simulink model "pump_elastic_sim"  (R2020a)
settings: Solver=VariableStepAuto  StartTime=0.0  StopTime=10  RelTol=1e-3
values from neighbouring files (symbols this model uses):
  A = 0.3    [Shape_Function.m]
  l = 8    [Shape_Function.m]
  rho = 7833    [Shape_Function.m]
undefined symbols (not defined in the file or in its folder): Al, B, Cd, Cl, g, G1, G2, G3, G4, G5, G6, h, Jx, Jy, K, m, mu0, Nr, P1, P2, P3, P4, P5, P6, PHI12, PHI20, PHI4, phi_init, PHIc, PHIf, PHIr, qv_init, R, radius, Ss, theta_init, vqv_init, Vref, vx, w, xA, xB, xdot_ref, xe, yB, zA, zB, zi_rip
settings Model: Creator=adelina  LastModifiedBy=Federico

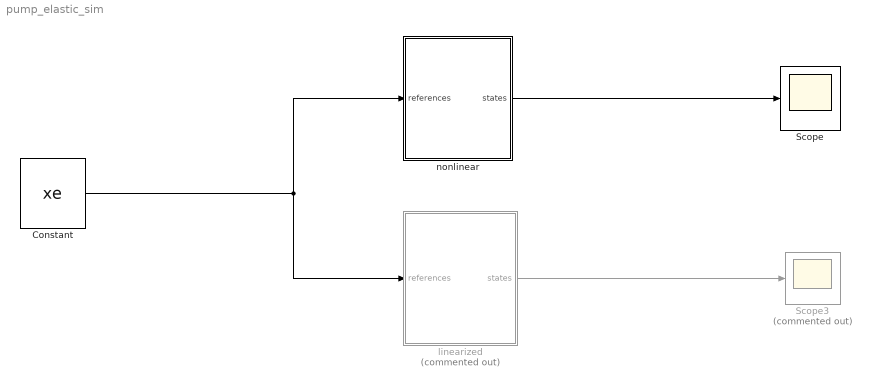
== system pump_elastic_sim ==
  Constant : Constant  Value=xe
  Scope : Scope
  Scope3 : Scope  Commented=on
  linearized : Subsystem  Commented=on
  nonlinear : Subsystem
  wires:
  linearized/1(states) -> Scope3/1
  nonlinear/1(states) -> Scope/1
  Constant/1 -> nonlinear/1(references), linearized/1(references)

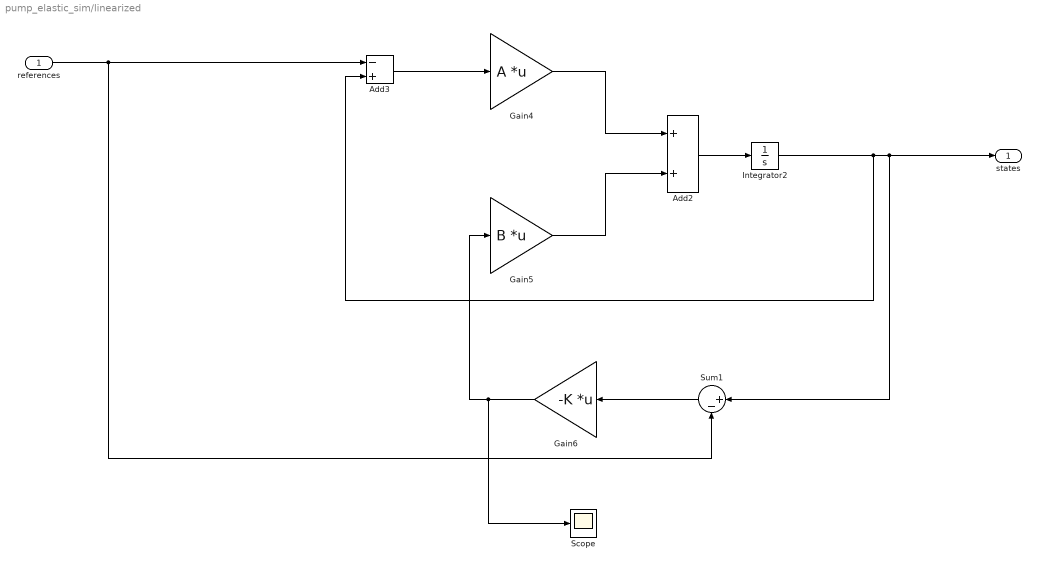
== system pump_elastic_sim/linearized ==
  references : Inport
  Add2 : Sum
  Add3 : Sum  Inputs=-+
  Gain4 : Gain  Gain=A  Multiplication=Matrix(K*u)
  Gain5 : Gain  Gain=B  Multiplication=Matrix(K*u)
  Gain6 : Gain  Gain=-K  Multiplication=Matrix(K*u)
  Integrator2 : Integrator  InitialCondition=[h;0;0;0;0;0;0;0;0;0;0;0]
  Scope : Scope
  Sum1 : Sum  Inputs=|+-
  states : Outport
  wires:
  Add2/1 -> Integrator2/1
  Gain5/1 -> Add2/2
  Gain6/1 -> Scope/1, Gain5/1
  Gain4/1 -> Add2/1
  Integrator2/1 -> states/1, Sum1/1, Add3/2
  Add3/1 -> Gain4/1
  references/1 -> Sum1/2, Add3/1
  Sum1/1 -> Gain6/1

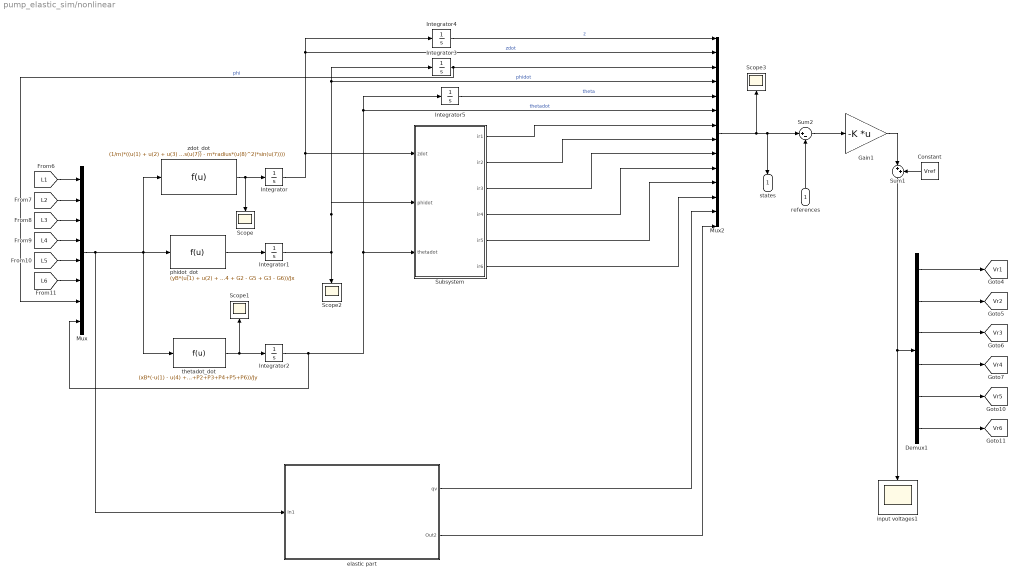
== system pump_elastic_sim/nonlinear ==
  references : Inport
  Constant : Constant  Value=Vref
  Demux1 : Demux  Outputs=6
  Gain1 : Gain  Gain=-K  Multiplication=Matrix(K*u)
  Integrator : Integrator
  Integrator1 : Integrator
  Integrator2 : Integrator
  Integrator3 : Integrator  InitialCondition=phi_init
  Integrator4 : Integrator  InitialCondition=h
  Integrator5 : Integrator  InitialCondition=theta_init
  Mux : Mux  Inputs=8
  Mux2 : Mux  Inputs=14
  Scope{,1..3} (4 alike) : Scope
  Subsystem : Subsystem
  Sum1 : Sum  Inputs=|++
  Sum2 : Sum  Inputs=|+-
  elastic part : Subsystem
  input voltages1 : Scope
  phidot_dot : Fcn  Expr=(yB*(u(1) + u(2) + u(3) - u(4) - u(5) - u(6)) + zB*(G1 - G4 + G2 - G5 + G3 - G6))/Jx
  thetadot_dot : Fcn  Expr=(xB*(-u(1) - u(4) + u(3) + u(6)) -zA*(rho*Ss*Cd/2)*(xdot_ref)^2+xA*(rho*Ss*Cl/2)*(xdot_ref)^2+zB*(P1+P2+P3+P4+P5+P6))/Jy
  zdot_dot : Fcn  Expr=(1/m)*((u(1) + u(2) + u(3) + u(4) + u(5) + u(6) - (rho*Ss*Cl/2)*(xdot_ref)^2 - m*g*cos(u(7)) - m*radius*(u(8)^2)*sin(u(7))))
  states : Outport
  tag scope: Vr1=global, Vr2=global, Vr3=global, Vr4=global, Vr5=global, Vr6=global
  wires:
  Mux/1 -> elastic part/1(In1), thetadot_dot/1, phidot_dot/1, zdot_dot/1
  zdot_dot/1 -> Scope/1, Integrator/1
  Integrator/1 -> Integrator4/1, Mux2/2, Subsystem/1(zdot)  "zdot"
  phidot_dot/1 -> Integrator1/1
  Integrator1/1 -> Scope2/1, Mux2/4, Integrator3/1, Subsystem/2(phidot)  "phidot"
  thetadot_dot/1 -> Integrator2/1, Scope1/1
  Integrator2/1 -> Mux2/6, Integrator5/1, Subsystem/3(thetadot), Mux/8  "thetadot"
  [L1] -> Mux/1
  [L2] -> Mux/2
  [L3] -> Mux/3
  [L4] -> Mux/4
  [L5] -> Mux/5
  [L6] -> Mux/6
  Integrator3/1 -> Mux2/3, Mux/7  "phi"
  Demux1/4 -> [Vr4]
  Demux1/3 -> [Vr3]
  Demux1/2 -> [Vr2]
  Demux1/1 -> [Vr1]
  Sum2/1 -> Gain1/1
  Demux1/5 -> [Vr5]
  Demux1/6 -> [Vr6]
  Integrator4/1 -> Mux2/1  "z"
  Integrator5/1 -> Mux2/5  "theta"
  Subsystem/1(ir1) -> Mux2/7
  Subsystem/2(ir2) -> Mux2/8
  Subsystem/3(ir3) -> Mux2/9
  Subsystem/4(ir4) -> Mux2/10
  Subsystem/5(ir5) -> Mux2/11
  Subsystem/6(ir6) -> Mux2/12
  Mux2/1 -> Scope3/1, states/1, Sum2/1
  elastic part/1(qv) -> Mux2/13
  elastic part/2(Out2) -> Mux2/14
  references/1 -> Sum2/2
  Gain1/1 -> Sum1/1
  Sum1/1 -> Demux1/1, input voltages1/1
  Constant/1 -> Sum1/2

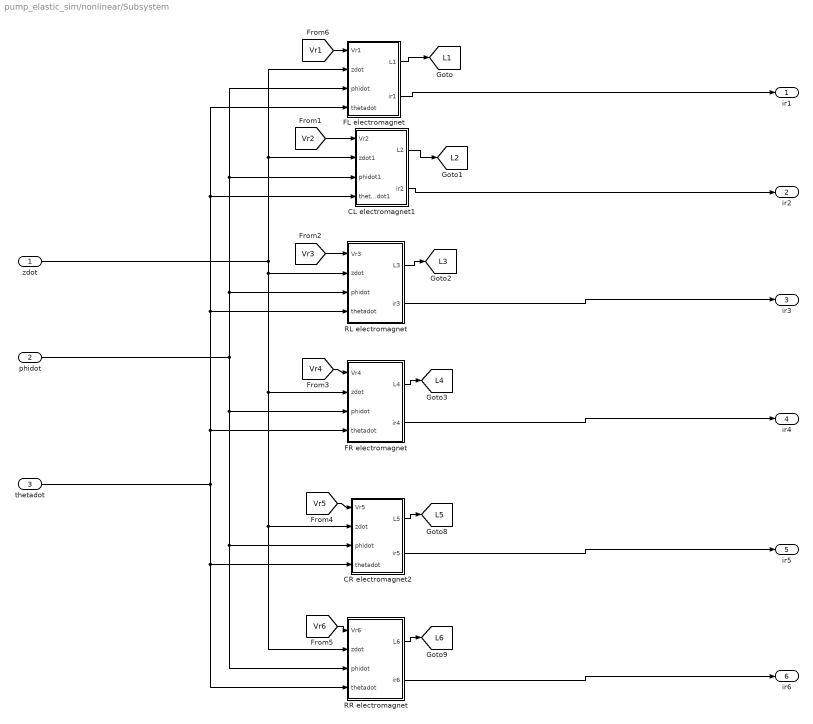
== system pump_elastic_sim/nonlinear/Subsystem ==
  zdot : Inport
  phidot : Inport  Port=2
  thetadot : Inport  Port=3
  CL electromagnet1 : Subsystem
  CR electromagnet2 : Subsystem
  FL electromagnet : Subsystem
  FR electromagnet : Subsystem
  RL electromagnet : Subsystem
  RR electromagnet : Subsystem
  ir1 : Outport
  ir2 : Outport  Port=2
  ir3 : Outport  Port=3
  ir4 : Outport  Port=4
  ir5 : Outport  Port=5
  ir6 : Outport  Port=6
  tag scope: L1=global, L2=global, L3=global, L4=global, L5=global, L6=global
  wires:
  CL electromagnet1/2(ir2) -> ir2/1
  [Vr3] -> RL electromagnet/1(Vr3)
  FR electromagnet/1(L4) -> [L4]
  CL electromagnet1/1(L2) -> [L2]
  FL electromagnet/1(L1) -> [L1]
  RR electromagnet/1(L6) -> [L6]
  CR electromagnet2/1(L5) -> [L5]
  [Vr6] -> RR electromagnet/1(Vr6)
  phidot/1 -> FR electromagnet/3(phidot), RR electromagnet/3(phidot), CR electromagnet2/3(phidot), FL electromagnet/3(phidot), CL electromagnet1/3(phidot1), RL electromagnet/3(phidot)
  [Vr4] -> FR electromagnet/1(Vr4)
  FR electromagnet/2(ir4) -> ir4/1
  zdot/1 -> CL electromagnet1/2(zdot1), FL electromagnet/2(zdot), RL electromagnet/2(zdot), FR electromagnet/2(zdot), RR electromagnet/2(zdot), CR electromagnet2/2(zdot)
  RL electromagnet/2(ir3) -> ir3/1
  FL electromagnet/2(ir1) -> ir1/1
  [Vr2] -> CL electromagnet1/1(Vr2)
  thetadot/1 -> RR electromagnet/4(thetadot), CR electromagnet2/4(thetadot), FL electromagnet/4(thetadot), CL electromagnet1/4(thetadot1), RL electromagnet/4(thetadot), FR electromagnet/4(thetadot)
  CR electromagnet2/2(ir5) -> ir5/1
  [Vr5] -> CR electromagnet2/1(Vr5)
  RR electromagnet/2(ir6) -> ir6/1
  RL electromagnet/1(L3) -> [L3]
  [Vr1] -> FL electromagnet/1(Vr1)

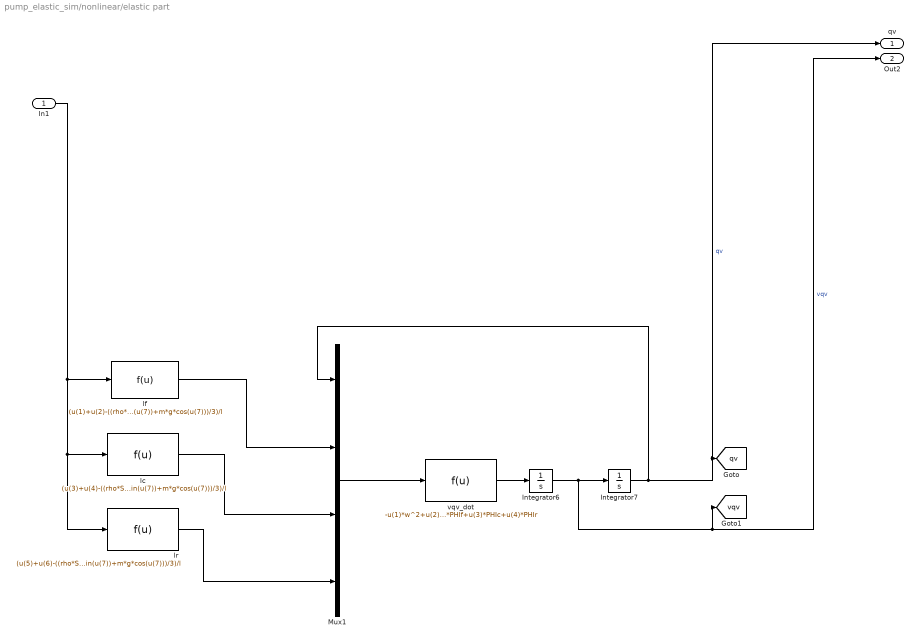
== system pump_elastic_sim/nonlinear/elastic part ==
  In1 : Inport
  Integrator6 : Integrator  InitialCondition=vqv_init
  Integrator7 : Integrator  InitialCondition=qv_init
  Mux1 : Mux
  lc : Fcn  Expr=(u(3)+u(4)-((rho*Ss*Cl/2)*(vx)^2+m*R*(u(8)^2)*sin(u(7))+m*g*cos(u(7)))/3)/l
  lf : Fcn  Expr=(u(1)+u(2)-((rho*Ss*Cl/2)*(vx)^2+m*R*(u(8)^2)*sin(u(7))+m*g*cos(u(7)))/3)/l
  lr : Fcn  Expr=(u(5)+u(6)-((rho*Ss*Cl/2)*(vx)^2+m*R*(u(8)^2)*sin(u(7))+m*g*cos(u(7)))/3)/l
  vqv_dot : Fcn  Expr=-u(1)*w^2+u(2)*PHIf+u(3)*PHIc+u(4)*PHIr
  qv : Outport
  Out2 : Outport  Port=2
  tag scope: qv=global, vqv=global
  wires:
  In1/1 -> lc/1, lr/1, lf/1
  Mux1/1 -> vqv_dot/1
  lf/1 -> Mux1/2
  vqv_dot/1 -> Integrator6/1
  Integrator7/1 -> qv/1, [qv], Mux1/1  "qv"
  lc/1 -> Mux1/3
  Integrator6/1 -> Out2/1, [vqv], Integrator7/1  "vqv"
  lr/1 -> Mux1/4

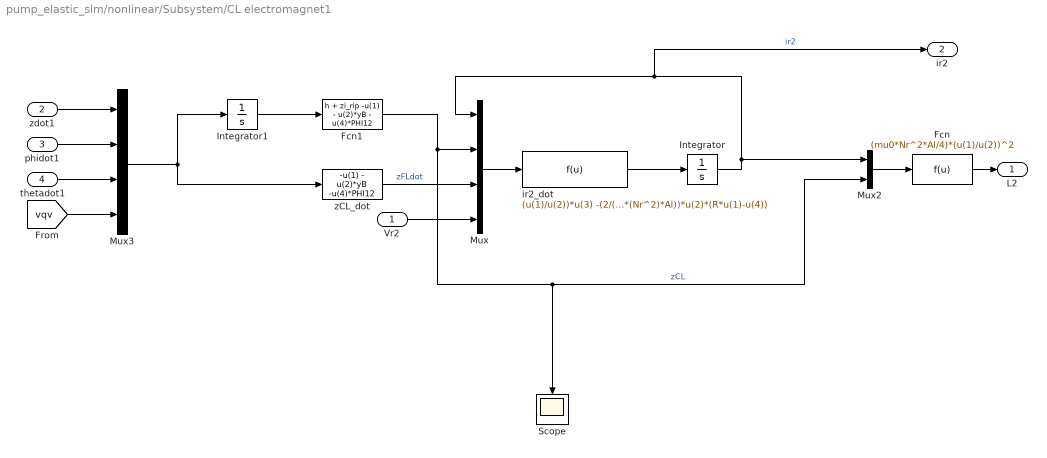
== system pump_elastic_sim/nonlinear/Subsystem/CL electromagnet1 ==
  Vr2 : Inport
  zdot1 : Inport  Port=2
  phidot1 : Inport  Port=3
  thetadot1 : Inport  Port=4
  Fcn : Fcn  Expr=(mu0*Nr^2*Al/4)*(u(1)/u(2))^2
  Fcn1 : Fcn  Expr=h + zi_rip -u(1) - u(2)*yB - u(4)*PHI12
  Integrator : Integrator
  Integrator1 : Integrator  InitialCondition=[h; phi_init; theta_init;qv_init]
  Mux : Mux
  Mux2 : Mux  Inputs=2
  Mux3 : Mux
  Scope : Scope
  ir2_dot : Fcn  Expr=(u(1)/u(2))*u(3) -(2/(mu0*(Nr^2)*Al))*u(2)*(R*u(1)-u(4))
  zCL_dot : Fcn  Expr=-u(1) - u(2)*yB -u(4)*PHI12
  L2 : Outport
  ir2 : Outport  Port=2
  wires:
  Mux/1 -> ir2_dot/1
  Vr2/1 -> Mux/4
  ir2_dot/1 -> Integrator/1
  Integrator/1 -> Mux2/1, ir2/1, Mux/1  "ir2"
  zCL_dot/1 -> Mux/3  "zFLdot"
  Fcn1/1 -> Scope/1, Mux2/2, Mux/2  "zCL"
  Mux2/1 -> Fcn/1
  Fcn/1 -> L2/1
  Integrator1/1 -> Fcn1/1
  thetadot1/1 -> Mux3/3
  phidot1/1 -> Mux3/2
  zdot1/1 -> Mux3/1
  [vqv] -> Mux3/4
  Mux3/1 -> zCL_dot/1, Integrator1/1

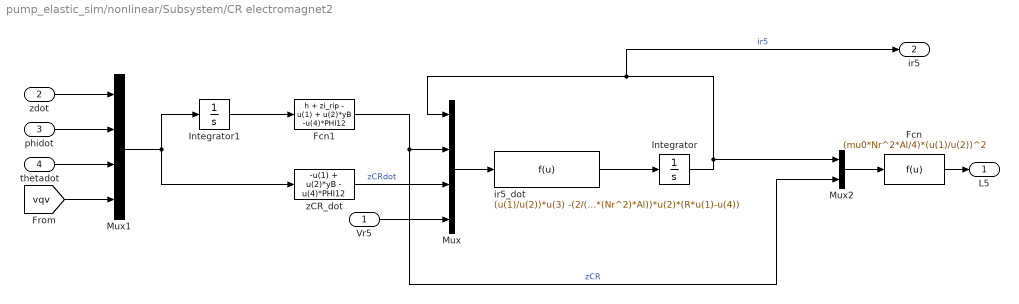
== system pump_elastic_sim/nonlinear/Subsystem/CR electromagnet2 ==
  Vr5 : Inport
  zdot : Inport  Port=2
  phidot : Inport  Port=3
  thetadot : Inport  Port=4
  Fcn : Fcn  Expr=(mu0*Nr^2*Al/4)*(u(1)/u(2))^2
  Fcn1 : Fcn  Expr=h + zi_rip - u(1) + u(2)*yB -u(4)*PHI12
  Integrator : Integrator
  Integrator1 : Integrator  InitialCondition=[h; phi_init; theta_init;qv_init]
  Mux : Mux
  Mux1 : Mux
  Mux2 : Mux  Inputs=2
  ir5_dot : Fcn  Expr=(u(1)/u(2))*u(3) -(2/(mu0*(Nr^2)*Al))*u(2)*(R*u(1)-u(4))
  zCR_dot : Fcn  Expr=-u(1) + u(2)*yB - u(4)*PHI12
  L5 : Outport
  ir5 : Outport  Port=2
  wires:
  Mux/1 -> ir5_dot/1
  Vr5/1 -> Mux/4
  ir5_dot/1 -> Integrator/1
  Integrator/1 -> Mux2/1, ir5/1, Mux/1  "ir5"
  zCR_dot/1 -> Mux/3  "zCRdot"
  Fcn1/1 -> Mux2/2, Mux/2  "zCR"
  Mux2/1 -> Fcn/1
  Fcn/1 -> L5/1
  Integrator1/1 -> Fcn1/1
  thetadot/1 -> Mux1/3
  phidot/1 -> Mux1/2
  zdot/1 -> Mux1/1
  [vqv] -> Mux1/4
  Mux1/1 -> Integrator1/1, zCR_dot/1

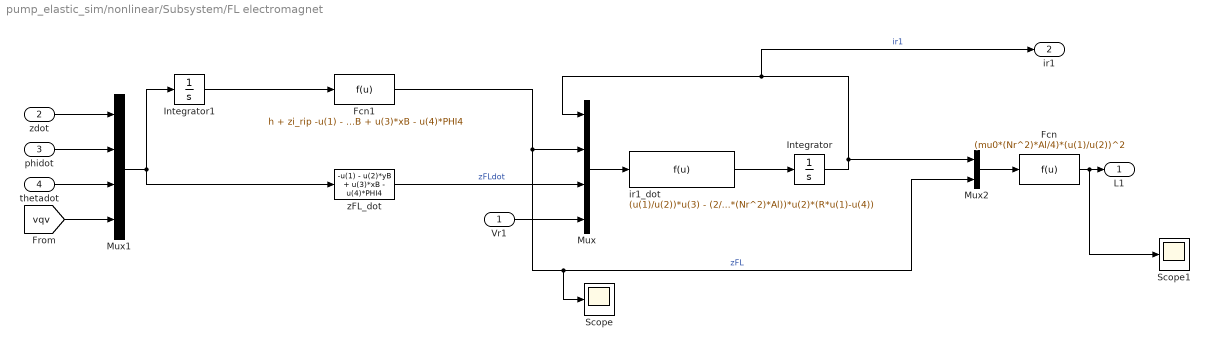
== system pump_elastic_sim/nonlinear/Subsystem/FL electromagnet ==
  Vr1 : Inport
  zdot : Inport  Port=2
  phidot : Inport  Port=3
  thetadot : Inport  Port=4
  Fcn : Fcn  Expr=(mu0*(Nr^2)*Al/4)*(u(1)/u(2))^2
  Fcn1 : Fcn  Expr=h + zi_rip -u(1) - u(2)*yB + u(3)*xB - u(4)*PHI4
  Integrator : Integrator
  Integrator1 : Integrator  InitialCondition=[h; phi_init; theta_init; qv_init]
  Mux : Mux
  Mux1 : Mux
  Mux2 : Mux  Inputs=2
  Scope : Scope
  Scope1 : Scope
  ir1_dot : Fcn  Expr=(u(1)/u(2))*u(3) - (2/(mu0*(Nr^2)*Al))*u(2)*(R*u(1)-u(4))
  zFL_dot : Fcn  Expr=-u(1) - u(2)*yB + u(3)*xB - u(4)*PHI4
  L1 : Outport
  ir1 : Outport  Port=2
  wires:
  Mux/1 -> ir1_dot/1
  Vr1/1 -> Mux/4
  ir1_dot/1 -> Integrator/1
  Integrator/1 -> Mux2/1, ir1/1, Mux/1  "ir1"
  Mux1/1 -> Integrator1/1, zFL_dot/1
  zdot/1 -> Mux1/1
  phidot/1 -> Mux1/2
  thetadot/1 -> Mux1/3
  zFL_dot/1 -> Mux/3  "zFLdot"
  Fcn1/1 -> Scope/1, Mux2/2, Mux/2  "zFL"
  Mux2/1 -> Fcn/1
  Fcn/1 -> Scope1/1, L1/1
  Integrator1/1 -> Fcn1/1
  [vqv] -> Mux1/4

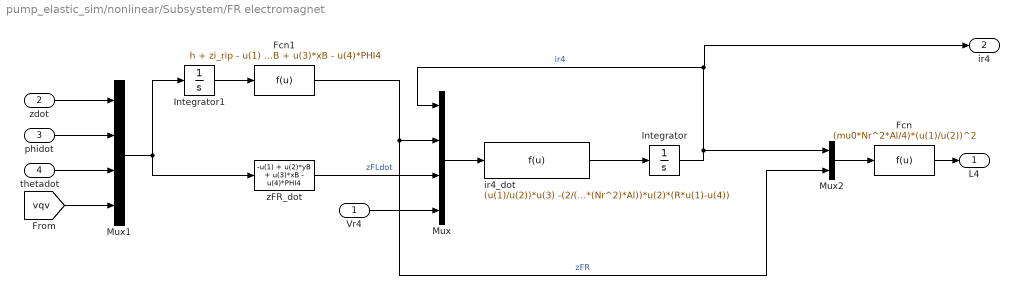
== system pump_elastic_sim/nonlinear/Subsystem/FR electromagnet ==
  Vr4 : Inport
  zdot : Inport  Port=2
  phidot : Inport  Port=3
  thetadot : Inport  Port=4
  Fcn : Fcn  Expr=(mu0*Nr^2*Al/4)*(u(1)/u(2))^2
  Fcn1 : Fcn  Expr=h + zi_rip - u(1) + u(2)*yB + u(3)*xB - u(4)*PHI4
  Integrator : Integrator
  Integrator1 : Integrator  InitialCondition=[h; phi_init; theta_init;qv_init]
  Mux : Mux
  Mux1 : Mux
  Mux2 : Mux  Inputs=2
  ir4_dot : Fcn  Expr=(u(1)/u(2))*u(3) -(2/(mu0*(Nr^2)*Al))*u(2)*(R*u(1)-u(4))
  zFR_dot : Fcn  Expr=-u(1) + u(2)*yB + u(3)*xB - u(4)*PHI4
  L4 : Outport
  ir4 : Outport  Port=2
  wires:
  Mux/1 -> ir4_dot/1
  Vr4/1 -> Mux/4
  ir4_dot/1 -> Integrator/1
  zFR_dot/1 -> Mux/3  "zFLdot"
  Fcn1/1 -> Mux2/2, Mux/2  "zFR"
  Mux2/1 -> Fcn/1
  Fcn/1 -> L4/1
  Integrator/1 -> Mux2/1, ir4/1, Mux/1  "ir4"
  Integrator1/1 -> Fcn1/1
  thetadot/1 -> Mux1/3
  phidot/1 -> Mux1/2
  zdot/1 -> Mux1/1
  [vqv] -> Mux1/4
  Mux1/1 -> zFR_dot/1, Integrator1/1

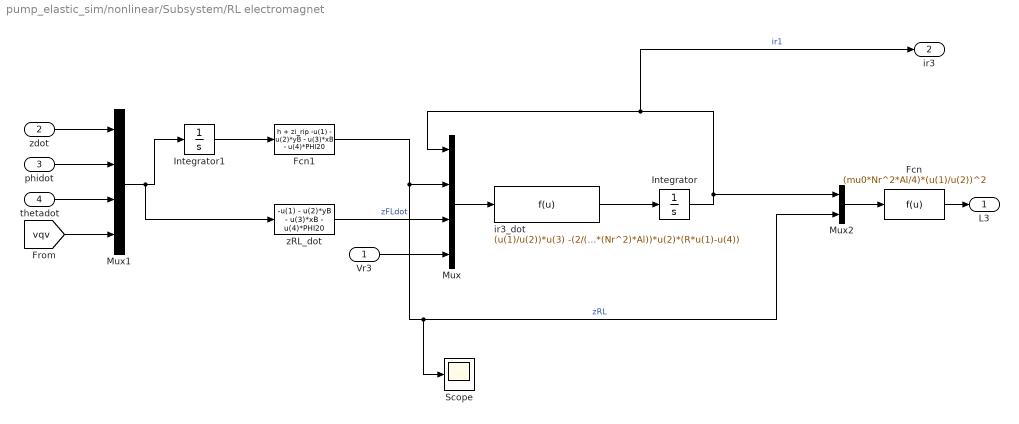
== system pump_elastic_sim/nonlinear/Subsystem/RL electromagnet ==
  Vr3 : Inport
  zdot : Inport  Port=2
  phidot : Inport  Port=3
  thetadot : Inport  Port=4
  Fcn : Fcn  Expr=(mu0*Nr^2*Al/4)*(u(1)/u(2))^2
  Fcn1 : Fcn  Expr=h + zi_rip -u(1) - u(2)*yB - u(3)*xB - u(4)*PHI20
  Integrator : Integrator
  Integrator1 : Integrator  InitialCondition=[h; phi_init; theta_init;qv_init]
  Mux : Mux
  Mux1 : Mux
  Mux2 : Mux  Inputs=2
  Scope : Scope
  ir3_dot : Fcn  Expr=(u(1)/u(2))*u(3) -(2/(mu0*(Nr^2)*Al))*u(2)*(R*u(1)-u(4))
  zRL_dot : Fcn  Expr=-u(1) - u(2)*yB - u(3)*xB - u(4)*PHI20
  L3 : Outport
  ir3 : Outport  Port=2
  wires:
  Mux/1 -> ir3_dot/1
  Vr3/1 -> Mux/4
  ir3_dot/1 -> Integrator/1
  zRL_dot/1 -> Mux/3  "zFLdot"
  Fcn1/1 -> Scope/1, Mux2/2, Mux/2  "zRL"
  Mux2/1 -> Fcn/1
  Fcn/1 -> L3/1
  Integrator/1 -> Mux2/1, ir3/1, Mux/1  "ir1"
  Integrator1/1 -> Fcn1/1
  thetadot/1 -> Mux1/3
  phidot/1 -> Mux1/2
  zdot/1 -> Mux1/1
  [vqv] -> Mux1/4
  Mux1/1 -> zRL_dot/1, Integrator1/1

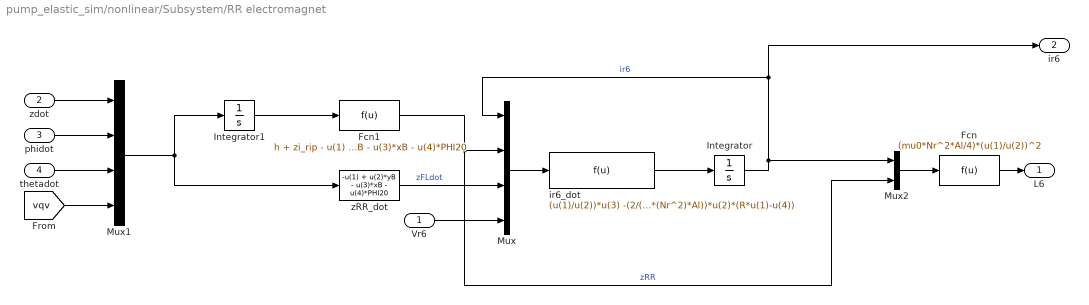
== system pump_elastic_sim/nonlinear/Subsystem/RR electromagnet ==
  Vr6 : Inport
  zdot : Inport  Port=2
  phidot : Inport  Port=3
  thetadot : Inport  Port=4
  Fcn : Fcn  Expr=(mu0*Nr^2*Al/4)*(u(1)/u(2))^2
  Fcn1 : Fcn  Expr=h + zi_rip - u(1) + u(2)*yB - u(3)*xB - u(4)*PHI20
  Integrator : Integrator
  Integrator1 : Integrator  InitialCondition=[h; phi_init; theta_init;qv_init]
  Mux : Mux
  Mux1 : Mux
  Mux2 : Mux  Inputs=2
  ir6_dot : Fcn  Expr=(u(1)/u(2))*u(3) -(2/(mu0*(Nr^2)*Al))*u(2)*(R*u(1)-u(4))
  zRR_dot : Fcn  Expr=-u(1) + u(2)*yB - u(3)*xB - u(4)*PHI20
  L6 : Outport
  ir6 : Outport  Port=2
  wires:
  Mux/1 -> ir6_dot/1
  Vr6/1 -> Mux/4
  ir6_dot/1 -> Integrator/1
  zRR_dot/1 -> Mux/3  "zFLdot"
  Fcn1/1 -> Mux2/2, Mux/2  "zRR"
  Mux2/1 -> Fcn/1
  Fcn/1 -> L6/1
  Integrator/1 -> Mux2/1, ir6/1, Mux/1  "ir6"
  Integrator1/1 -> Fcn1/1
  thetadot/1 -> Mux1/3
  phidot/1 -> Mux1/2
  zdot/1 -> Mux1/1
  [vqv] -> Mux1/4
  Mux1/1 -> Integrator1/1, zRR_dot/1
